simulink model "pendulumExample"  (Simulink 7.3)
settings: Solver=ode3  StartTime=0.0  StopTime=tof  FixedStep=0.01  RelTol=1e-3
InitFcn:
  | init
StopFcn:
  | plotlab
values from neighbouring files (symbols this model uses):
  Arm = [0 1;-wn^2 -2*ksi*wn]    [init.m]    (also in initPendulum2.m)
  B = [0 1]'    [init.m]    (also in initPendulum2.m = [0 0 ; 0 1])
  Brm = [0 wn^2]'    [init.m]    (also in initPendulum2.m)
  epsilon = 0.08    [init.m]    (also in initPendulum2.m)
  GammaW = 3.5    [init.m]    (also in initPendulum2.m)
  K = [1.5 0;0 1.3]    [init.m]    (also in initPendulum2.m)
  p = 10    [init.m]
  P = lyap(A',Q)    [init.m]    (also in initPendulum2.m)
  r = 1    [init.m]
  tr = [20 25]    [init.m]
  W0 = [2 -0.5 1]'    [init.m]    (also in initPendulum2.m = [2 -0.5 1 ; 0 0 0]')
  x0 = [1 1]'    [init.m]    (also in initPendulum2.m)
libraries: simulink x2, dspbuff3 x1, dspmtrx3 x1
settings Model: Creator=Alp  LastModifiedBy=alp.marangoz

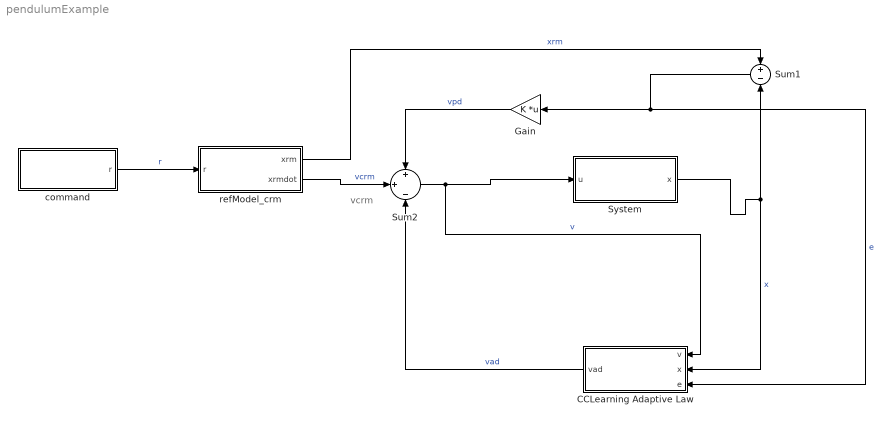
== system pendulumExample ==
  note: vcrm
  CCLearning Adaptive Law : Subsystem  TreatAsAtomicUnit=on
  Gain : Gain  Gain=K  Multiplication=Matrix(K*u)  ParameterDataType=fixdt(1, 16)  ParameterScaling=2^0  OutDataType=fixdt(1, 16)  OutScaling=2^0
  Sum1 : Sum  Inputs=+|-  OutDataType=fixdt(1, 16)  OutScaling=2^0
  Sum2 : Sum  Inputs=+|+|-  OutDataType=fixdt(1, 16)  OutScaling=2^0
  System : Subsystem  TreatAsAtomicUnit=on
  command : Subsystem
  refModel_crm : Subsystem  TreatAsAtomicUnit=on
  wires:
  command/1(r) -> refModel_crm/1(r)  "r"
  refModel_crm/1(xrm) -> Sum1/1  "xrm"
  Sum1/1 -> Gain/1, CCLearning Adaptive Law/3(e)  "e"
  Gain/1 -> Sum2/1  "vpd"
  refModel_crm/2(xrmdot) -> Sum2/2  "vcrm"
  Sum2/1 -> System/1(u), CCLearning Adaptive Law/1(v)  "v"
  CCLearning Adaptive Law/1(vad) -> Sum2/3  "vad"
  System/1(x) -> Sum1/2, CCLearning Adaptive Law/2(x)  "x"

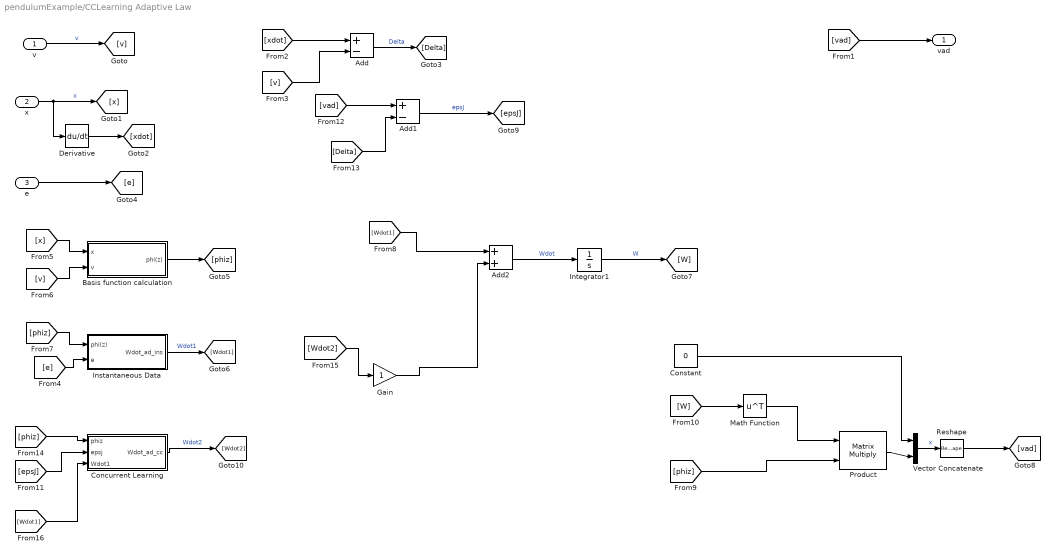
== system pendulumExample/CCLearning Adaptive Law ==
  v : Inport  OutDataType=fixdt(1, 16)  OutScaling=2^0
  x : Inport  Port=2  OutDataType=fixdt(1, 16)  OutScaling=2^0
  e : Inport  Port=3  OutDataType=fixdt(1, 16)  OutScaling=2^0
  Add : Sum  Inputs=+-  OutDataType=fixdt(1, 16)  OutScaling=2^-10
  Add1 : Sum  Inputs=+-  OutDataType=fixdt(1, 16)  OutScaling=2^-10
  Add2 : Sum  OutDataType=fixdt(1, 16)  OutScaling=2^-10
  Basis function calculation : Subsystem  TreatAsAtomicUnit=on
  Concurrent Learning : Subsystem  TreatAsAtomicUnit=on
  Constant : Constant  Value=0  OutDataType=fixdt(1, 16)  OutScaling=2^0
  Derivative : Derivative
  Gain : Gain  ParameterDataType=fixdt(1, 16)  ParameterScaling=2^0  OutDataType=fixdt(1, 16)  OutScaling=2^0
  Instantaneous Data : Subsystem  TreatAsAtomicUnit=on
  Integrator1 : Integrator  InitialCondition=W0
  Math Function : Math  Operator=transpose  OutDataType=fixdt(1, 16)  OutScaling=2^0  SaturateOnIntegerOverflow=on
  Product : Product  Multiplication=Matrix(*)  OutDataType=fixdt(1, 16)  OutScaling=2^0  RndMeth=Zero
  Reshape : Reshape  OutputDimensionality=Column vector (2-D)
  Vector Concatenate : Concatenate  Mode=Vector
  vad : Outport  OutDataType=fixdt(1, 16)  OutScaling=2^0
  wires:
  v/1 -> [v]  "v"
  [vad] -> vad/1
  x/1 -> [x], Derivative/1  "x"
  Derivative/1 -> [xdot]
  [xdot] -> Add/1
  [v] -> Add/2
  Add/1 -> [Delta]  "Delta"
  e/1 -> [e]
  [e] -> Instantaneous Data/2(e)
  [x] -> Basis function calculation/1(x)
  [v] -> Basis function calculation/2(v)
  Basis function calculation/1(phi(z)) -> [phiz]
  [phiz] -> Instantaneous Data/1(phi(z))
  Instantaneous Data/1(Wdot_ad_ins) -> [Wdot1]  "Wdot1"
  Integrator1/1 -> [W]  "W"
  [W] -> Math Function/1
  Math Function/1 -> Product/1
  [phiz] -> Product/2
  Vector Concatenate/1 -> Reshape/1  "x"
  Product/1 -> Vector Concatenate/2
  Reshape/1 -> [vad]
  Constant/1 -> Vector Concatenate/1
  [vad] -> Add1/1
  [Delta] -> Add1/2
  Add1/1 -> [epsJ]  "epsJ"
  [phiz] -> Concurrent Learning/1(phiz)
  Concurrent Learning/1(Wdot_ad_cc) -> [Wdot2]  "Wdot2"
  [epsJ] -> Concurrent Learning/2(epsj)
  [Wdot1] -> Add2/1
  Add2/1 -> Integrator1/1  "Wdot"
  [Wdot2] -> Gain/1
  [Wdot1] -> Concurrent Learning/3(Wdot1)
  Gain/1 -> Add2/2

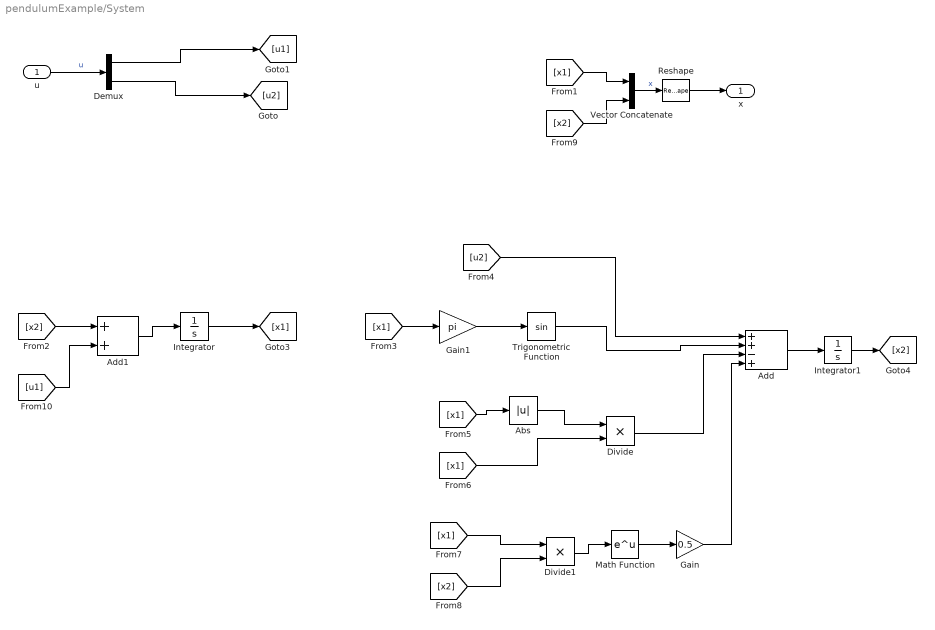
== system pendulumExample/System ==
  u : Inport  OutDataType=fixdt(1, 16)  OutScaling=2^0
  Abs : Abs  OutDataType=fixdt(1, 16)  OutScaling=2^0
  Add : Sum  Inputs=++-+  OutDataType=fixdt(1, 16)  OutScaling=2^-10
  Add1 : Sum  OutDataType=fixdt(1, 16)  OutScaling=2^-10
  Demux : Demux  Outputs=2
  Divide : Product  Inputs=**  OutDataType=fixdt(1, 16)  OutScaling=2^-10
  Divide1 : Product  Inputs=**  OutDataType=fixdt(1, 16)  OutScaling=2^-10
  Gain : Gain  Gain=0.5  ParameterDataType=fixdt(1, 16)  ParameterScaling=2^0  OutDataType=fixdt(1, 16)  OutScaling=2^0
  Gain1 : Gain  Gain=pi  ParameterDataType=fixdt(1, 16)  ParameterScaling=2^0  OutDataType=fixdt(1, 16)  OutScaling=2^0
  Integrator : Integrator  InitialCondition=x0(1,1)
  Integrator1 : Integrator  InitialCondition=x0(2,1)
  Math Function : Math  OutDataType=fixdt(1, 16)  OutScaling=2^0  SaturateOnIntegerOverflow=on
  Reshape : Reshape  OutputDimensionality=Column vector (2-D)
  Trigonometric Function : Trigonometry
  Vector Concatenate : Concatenate  Mode=Vector
  x : Outport  OutDataType=fixdt(1, 16)  OutScaling=2^0
  wires:
  Integrator/1 -> [x1]
  [x1] -> Gain1/1
  [x1] -> Abs/1
  Abs/1 -> Divide/1
  [x1] -> Divide/2
  [x1] -> Divide1/1
  [x2] -> Divide1/2
  Divide1/1 -> Math Function/1
  Math Function/1 -> Gain/1
  [u2] -> Add/1
  Trigonometric Function/1 -> Add/2
  Divide/1 -> Add/3
  Gain/1 -> Add/4
  Add/1 -> Integrator1/1
  Integrator1/1 -> [x2]
  [x1] -> Vector Concatenate/1
  [x2] -> Vector Concatenate/2
  Vector Concatenate/1 -> Reshape/1  "x"
  Reshape/1 -> x/1
  u/1 -> Demux/1  "u"
  Demux/1 -> [u1]
  Demux/2 -> [u2]
  Gain1/1 -> Trigonometric Function/1
  [x2] -> Add1/1
  Add1/1 -> Integrator/1
  [u1] -> Add1/2

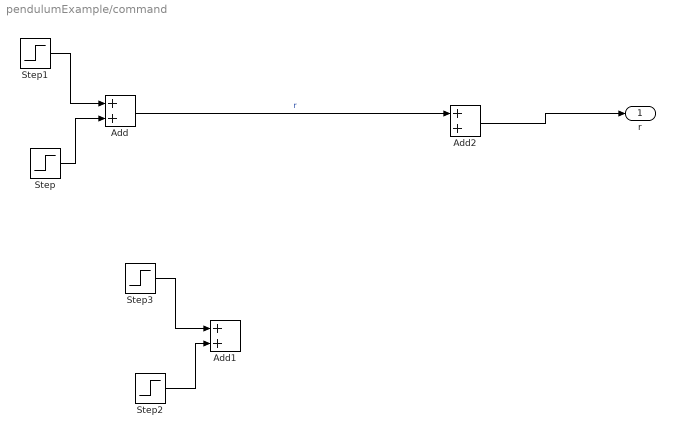
== system pendulumExample/command ==
  Add : Sum  OutDataType=fixdt(1, 16)  OutScaling=2^-10
  Add1 : Sum  OutDataType=fixdt(1, 16)  OutScaling=2^-10
  Add2 : Sum  OutDataType=fixdt(1, 16)  OutScaling=2^-10
  Step : Step  Time=tr(2)  After=-r  SampleTime=0
  Step1 : Step  Time=tr(1)  After=r  SampleTime=0
  Step2 : Step  Time=45  After=-r  SampleTime=0
  Step3 : Step  Time=40  After=r  SampleTime=0
  r : Outport
  wires:
  Step1/1 -> Add/1
  Step/1 -> Add/2
  Step3/1 -> Add1/1
  Step2/1 -> Add1/2
  Add/1 -> Add2/1  "r"
  Add2/1 -> r/1

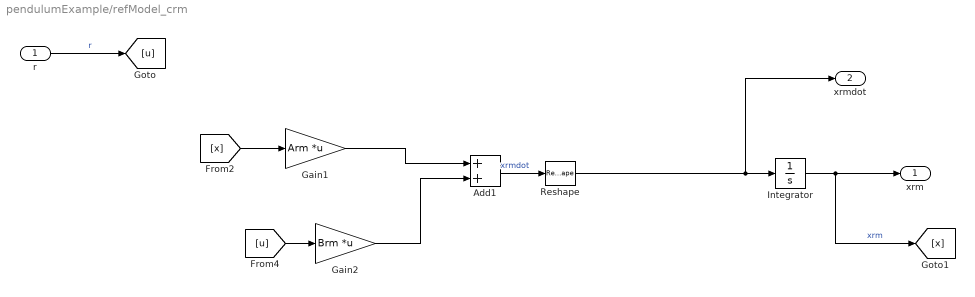
== system pendulumExample/refModel_crm ==
  r : Inport  OutDataType=fixdt(1, 16)  OutScaling=2^0
  Add1 : Sum  OutDataType=fixdt(1, 16)  OutScaling=2^-10
  Gain1 : Gain  Gain=Arm  Multiplication=Matrix(K*u)  ParameterDataType=fixdt(1, 16)  ParameterScaling=2^0  OutDataType=fixdt(1, 16)  OutScaling=2^0
  Gain2 : Gain  Gain=Brm  Multiplication=Matrix(K*u)  ParameterDataType=fixdt(1, 16)  ParameterScaling=2^0  OutDataType=fixdt(1, 16)  OutScaling=2^0
  Integrator : Integrator  InitialCondition=x0
  Reshape : Reshape  OutputDimensionality=Column vector (2-D)
  xrm : Outport  OutDataType=fixdt(1, 16)  OutScaling=2^0
  xrmdot : Outport  Port=2  OutDataType=fixdt(1, 16)  OutScaling=2^0
  wires:
  [x] -> Gain1/1
  r/1 -> [u]  "r"
  [u] -> Gain2/1
  Gain1/1 -> Add1/1
  Gain2/1 -> Add1/2
  Add1/1 -> Reshape/1  "xrmdot"
  Integrator/1 -> xrm/1, [x]  "xrm"
  Reshape/1 -> Integrator/1, xrmdot/1

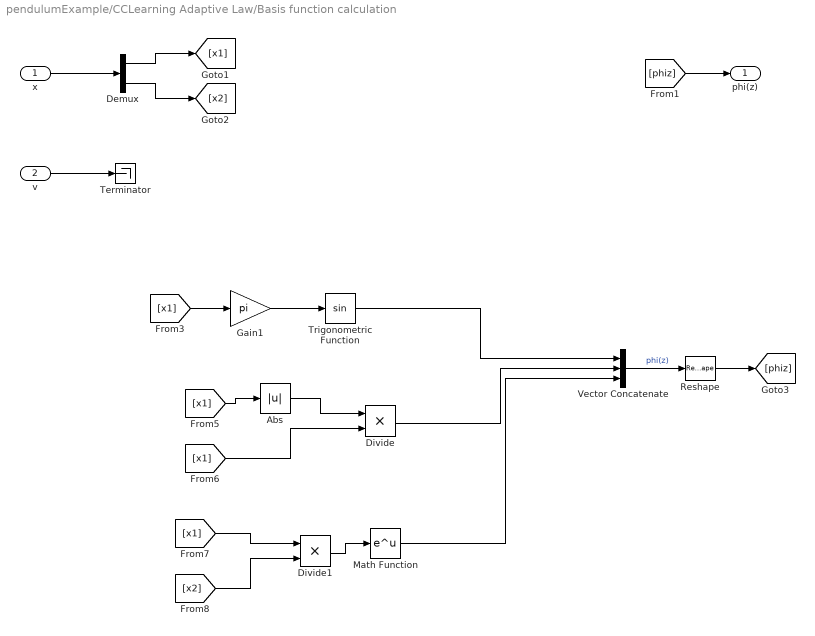
== system pendulumExample/CCLearning Adaptive Law/Basis function calculation ==
  x : Inport  OutDataType=fixdt(1, 16)  OutScaling=2^0
  v : Inport  Port=2  OutDataType=fixdt(1, 16)  OutScaling=2^0
  Abs : Abs  OutDataType=fixdt(1, 16)  OutScaling=2^0
  Demux : Demux  Outputs=2
  Divide : Product  Inputs=**  OutDataType=fixdt(1, 16)  OutScaling=2^-10
  Divide1 : Product  Inputs=**  OutDataType=fixdt(1, 16)  OutScaling=2^-10
  Gain1 : Gain  Gain=pi  ParameterDataType=fixdt(1, 16)  ParameterScaling=2^0  OutDataType=fixdt(1, 16)  OutScaling=2^0
  Math Function : Math  OutDataType=fixdt(1, 16)  OutScaling=2^0  SaturateOnIntegerOverflow=on
  Reshape : Reshape  OutputDimensionality=Column vector (2-D)
  Terminator : Terminator
  Trigonometric Function : Trigonometry
  Vector Concatenate : Concatenate  NumInputs=3  Mode=Vector
  phi(z) : Outport  OutDataType=fixdt(1, 16)  OutScaling=2^0
  wires:
  x/1 -> Demux/1
  v/1 -> Terminator/1
  [phiz] -> phi(z)/1
  [x1] -> Gain1/1
  [x1] -> Abs/1
  Abs/1 -> Divide/1
  [x1] -> Divide/2
  [x1] -> Divide1/1
  [x2] -> Divide1/2
  Divide1/1 -> Math Function/1
  Gain1/1 -> Trigonometric Function/1
  Demux/1 -> [x1]
  Demux/2 -> [x2]
  Vector Concatenate/1 -> Reshape/1  "phi(z)"
  Reshape/1 -> [phiz]
  Trigonometric Function/1 -> Vector Concatenate/1
  Divide/1 -> Vector Concatenate/2
  Math Function/1 -> Vector Concatenate/3

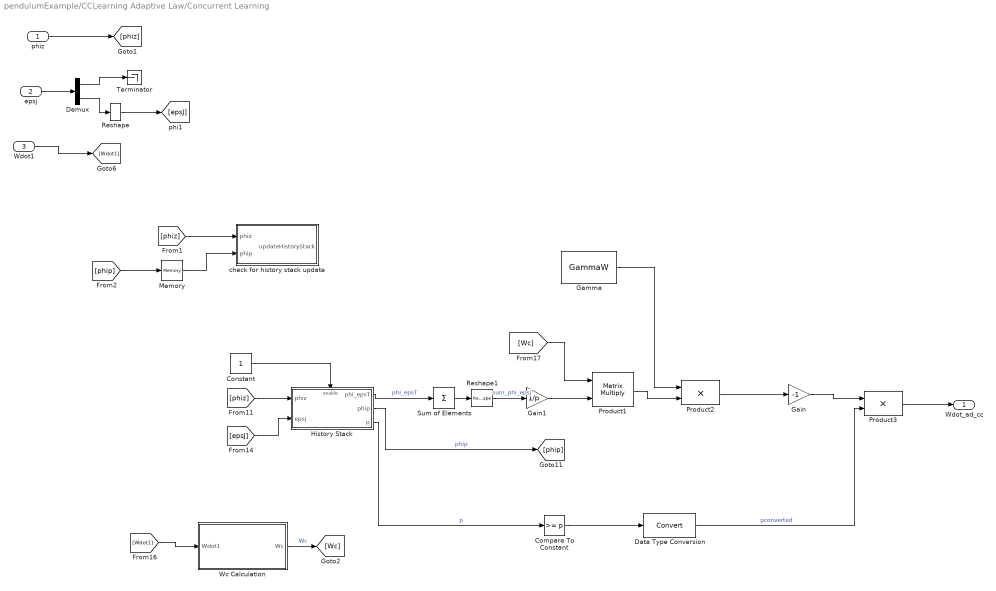
== system pendulumExample/CCLearning Adaptive Law/Concurrent Learning ==
  phiz : Inport  OutDataType=fixdt(1, 16)  OutScaling=2^0
  epsj : Inport  Port=2  OutDataType=fixdt(1, 16)  OutScaling=2^0
  Wdot1 : Inport  Port=3
  Compare To Constant : simulink/Logic and Bit Operations/Compare To Constant  SystemSampleTime=-1  relop=>=  const=p  LogicOutDataTypeMode=uint8  ZeroCross=off
  Constant : Constant  OutDataType=fixdt(1, 16)  OutScaling=2^0
  Data Type Conversion : DataTypeConversion  OutDataType=fixdt(1, 16)  OutScaling=2^0
  Demux : Demux  Outputs=2
  Gain : Gain  Gain=-1  ParameterDataType=fixdt(1, 16)  ParameterScaling=2^0  OutDataType=fixdt(1, 16)  OutScaling=2^0
  Gain1 : Gain  Gain=1/p  ParameterDataType=fixdt(1, 16)  ParameterScaling=2^0  OutDataType=fixdt(1, 16)  OutScaling=2^0
  Gamma : Constant  Value=GammaW  VectorParams1D=off  OutDataType=fixdt(1, 16)  OutScaling=2^0
  History Stack : Subsystem  TreatAsAtomicUnit=on
  Memory : Memory
  Product1 : Product  Multiplication=Matrix(*)  OutDataType=fixdt(1, 16)  OutScaling=2^0  RndMeth=Zero
  Product2 : Product  OutDataType=fixdt(1, 16)  OutScaling=2^0  RndMeth=Zero
  Product3 : Product  OutDataType=fixdt(1, 16)  OutScaling=2^0  RndMeth=Zero
  Reshape : Reshape  OutputDimensionality=Column vector (2-D)
  Reshape1 : Reshape  OutputDimensionality=Column vector (2-D)
  Sum of Elements : Sum  Inputs=+  CollapseMode=Specified dimension  OutDataType=fixdt(1, 16)  OutScaling=2^-10
  Terminator : Terminator
  Wc Calculation : Subsystem
  check for history stack update : Subsystem  TreatAsAtomicUnit=on
  Wdot_ad_cc : Outport  OutDataType=fixdt(1, 16)  OutScaling=2^0
  wires:
  [phiz] -> History Stack/1(phiz)
  [epsJ] -> History Stack/2(epsj)
  History Stack/1(phi_epsT) -> Sum of Elements/1  "phi_epsT"
  Gamma/1 -> Product2/1
  Product2/1 -> Gain/1
  History Stack/2(phip) -> [phip]  "phip"
  phiz/1 -> [phiz]
  Demux/1 -> Terminator/1
  Demux/2 -> Reshape/1
  epsj/1 -> Demux/1
  Reshape/1 -> [epsJ]
  [phiz] -> check for history stack update/1(phiz)
  [phip] -> Memory/1
  Memory/1 -> check for history stack update/2(phip)
  Sum of Elements/1 -> Reshape1/1
  Wdot1/1 -> [Wdot1]
  [Wdot1] -> Wc Calculation/1(Wdot1)
  Wc Calculation/1(Wc) -> [Wc]  "Wc"
  Reshape1/1 -> Gain1/1  "sum_phi_epsj"
  Product1/1 -> Product2/2
  [Wc] -> Product1/1
  Gain1/1 -> Product1/2
  History Stack/3(p) -> Compare To Constant/1  "p"
  Compare To Constant/1 -> Data Type Conversion/1
  Gain/1 -> Product3/1
  Data Type Conversion/1 -> Product3/2  "pconverted"
  Product3/1 -> Wdot_ad_cc/1
  Constant/1 -> History Stack/Enable

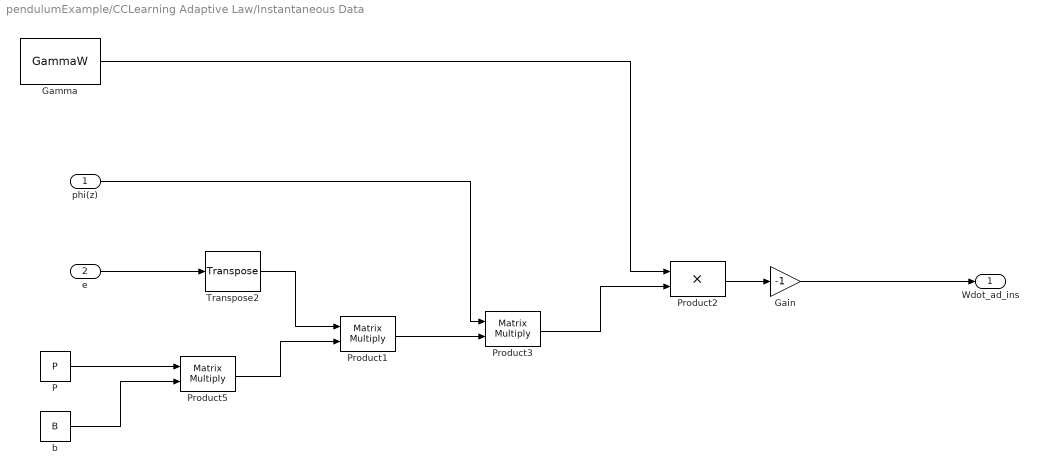
== system pendulumExample/CCLearning Adaptive Law/Instantaneous Data ==
  phi(z) : Inport  OutDataType=fixdt(1, 16)  OutScaling=2^0
  e : Inport  Port=2  OutDataType=fixdt(1, 16)  OutScaling=2^0
  Gain : Gain  Gain=-1  ParameterDataType=fixdt(1, 16)  ParameterScaling=2^0  OutDataType=fixdt(1, 16)  OutScaling=2^0
  Gamma : Constant  Value=GammaW  VectorParams1D=off  OutDataType=fixdt(1, 16)  OutScaling=2^0
  P : Constant  Value=P  VectorParams1D=off  OutDataType=fixdt(1, 16)  OutScaling=2^0
  Product1 : Product  Multiplication=Matrix(*)  OutDataType=fixdt(1, 16)  OutScaling=2^0  RndMeth=Zero
  Product2 : Product  OutDataType=fixdt(1, 16)  OutScaling=2^0  RndMeth=Zero
  Product3 : Product  Multiplication=Matrix(*)  OutDataType=fixdt(1, 16)  OutScaling=2^0  RndMeth=Zero
  Product5 : Product  Multiplication=Matrix(*)  OutDataType=fixdt(1, 16)  OutScaling=2^0  RndMeth=Zero
  Transpose2 : dspmtrx3/Transpose  SystemSampleTime=-1  Hermitian=off  overflowFlag=off
  b : Constant  Value=B  VectorParams1D=off  OutDataType=fixdt(1, 16)  OutScaling=2^0
  Wdot_ad_ins : Outport  OutDataType=fixdt(1, 16)  OutScaling=2^0
  wires:
  P/1 -> Product5/1
  b/1 -> Product5/2
  e/1 -> Transpose2/1
  Transpose2/1 -> Product1/1
  Product5/1 -> Product1/2
  phi(z)/1 -> Product3/1
  Product1/1 -> Product3/2
  Gamma/1 -> Product2/1
  Product3/1 -> Product2/2
  Product2/1 -> Gain/1
  Gain/1 -> Wdot_ad_ins/1

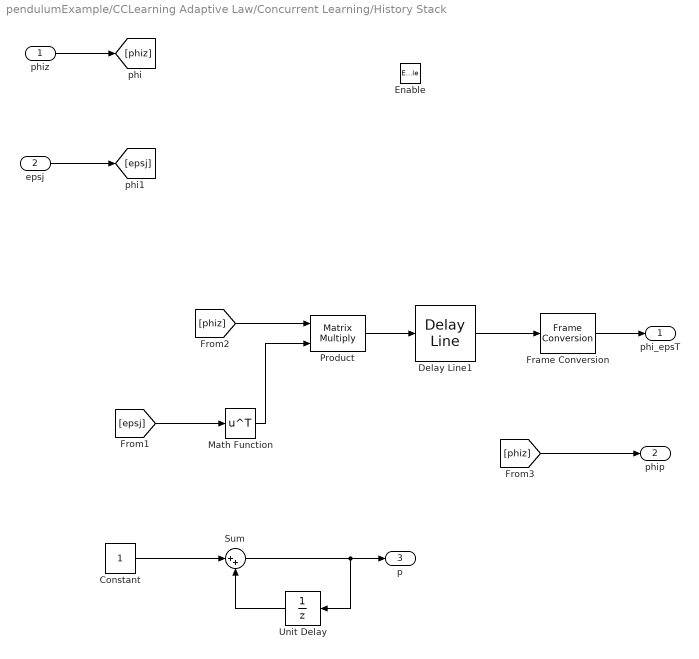
== system pendulumExample/CCLearning Adaptive Law/Concurrent Learning/History Stack ==
  phiz : Inport  OutDataType=fixdt(1, 16)  OutScaling=2^0
  epsj : Inport  Port=2  OutDataType=fixdt(1, 16)  OutScaling=2^0
  Enable : EnablePort
  Constant : Constant  OutDataType=fixdt(1, 16)  OutScaling=2^0
  Delay Line1 : dspbuff3/Delay Line  siz=p  ic=0  directfeed=on  enable_output=off  hold_output=off
  Frame Conversion : FrameConversion  OutFrame=Sample-based
  Math Function : Math  Operator=transpose  OutDataType=fixdt(1, 16)  OutScaling=2^0  SaturateOnIntegerOverflow=on
  Product : Product  Multiplication=Matrix(*)  OutDataType=fixdt(1, 16)  OutScaling=2^0  RndMeth=Zero
  Sum : Sum  Inputs=|++  OutDataType=fixdt(1, 16)  OutScaling=2^0
  Unit Delay : UnitDelay  SampleTime=-1
  phi_epsT : Outport  OutDataType=fixdt(1, 16)  OutScaling=2^0
  phip : Outport  Port=2  OutDataType=fixdt(1, 16)  OutScaling=2^0
  p : Outport  Port=3  OutDataType=fixdt(1, 16)  OutScaling=2^0
  wires:
  [phiz] -> Product/1
  phiz/1 -> [phiz]
  [epsj] -> Math Function/1
  Product/1 -> Delay Line1/1
  Delay Line1/1 -> Frame Conversion/1
  [phiz] -> phip/1
  Math Function/1 -> Product/2
  epsj/1 -> [epsj]
  Frame Conversion/1 -> phi_epsT/1
  Constant/1 -> Sum/1
  Sum/1 -> p/1, Unit Delay/1
  Unit Delay/1 -> Sum/2

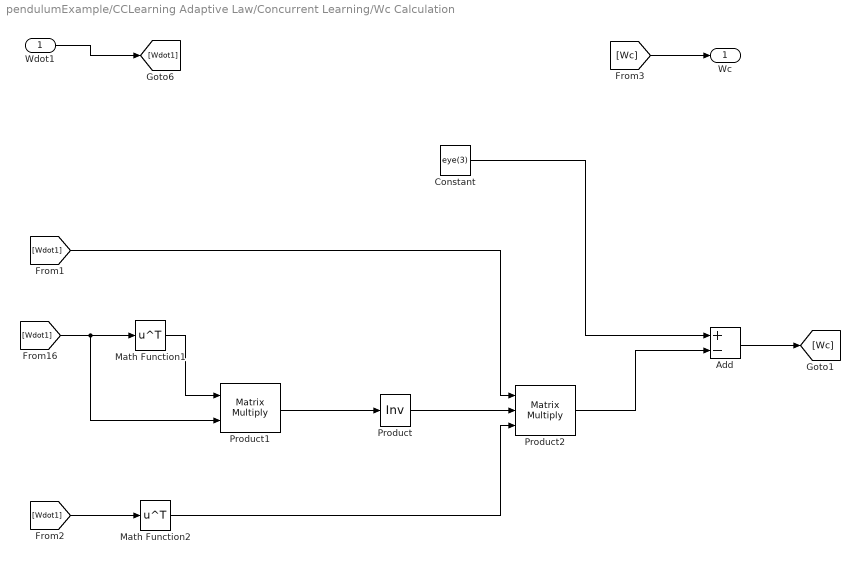
== system pendulumExample/CCLearning Adaptive Law/Concurrent Learning/Wc Calculation ==
  Wdot1 : Inport
  Add : Sum  Inputs=+-  OutDataType=fixdt(1, 16)  OutScaling=2^-10
  Constant : Constant  Value=eye(3)  OutDataType=fixdt(1, 16)  OutScaling=2^0
  Math Function1 : Math  Operator=transpose  OutDataType=fixdt(1, 16)  OutScaling=2^0  SaturateOnIntegerOverflow=on
  Math Function2 : Math  Operator=transpose  OutDataType=fixdt(1, 16)  OutScaling=2^0  SaturateOnIntegerOverflow=on
  Product : Product  Inputs=/  Multiplication=Matrix(*)  OutDataType=fixdt(1, 16)  OutScaling=2^0  RndMeth=Zero
  Product1 : Product  Multiplication=Matrix(*)  OutDataType=fixdt(1, 16)  OutScaling=2^0  RndMeth=Zero
  Product2 : Product  Inputs=***  Multiplication=Matrix(*)  OutDataType=fixdt(1, 16)  OutScaling=2^0  RndMeth=Zero
  Wc : Outport
  wires:
  [Wdot1] -> Math Function1/1, Product1/2
  Math Function1/1 -> Product1/1
  Product1/1 -> Product/1
  Wdot1/1 -> [Wdot1]
  [Wdot1] -> Math Function2/1
  [Wdot1] -> Product2/1
  Product/1 -> Product2/2
  Math Function2/1 -> Product2/3
  Constant/1 -> Add/1
  Add/1 -> [Wc]
  [Wc] -> Wc/1
  Product2/1 -> Add/2

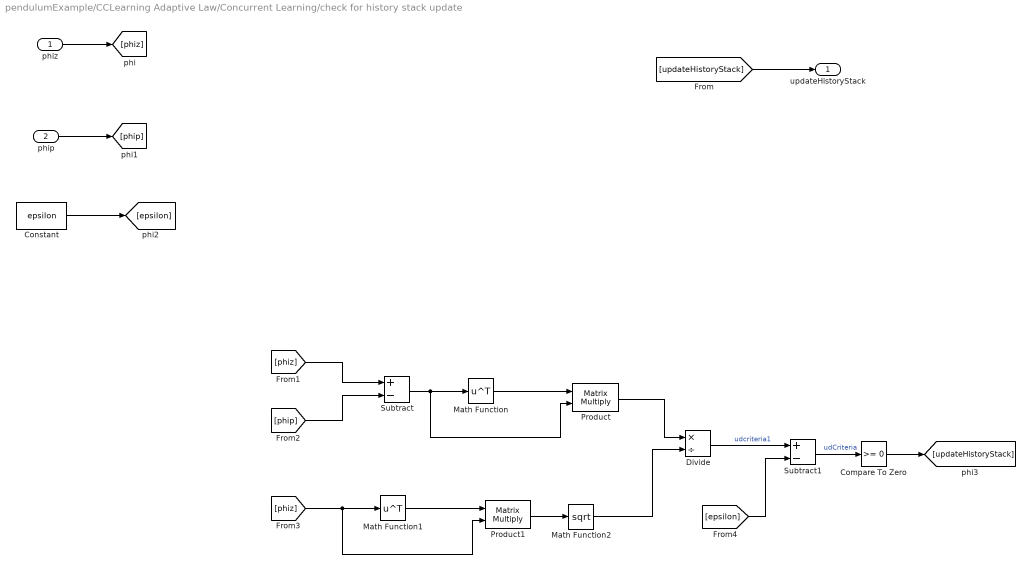
== system pendulumExample/CCLearning Adaptive Law/Concurrent Learning/check for history stack update ==
  phiz : Inport  OutDataType=fixdt(1, 16)  OutScaling=2^0
  phip : Inport  Port=2  OutDataType=fixdt(1, 16)  OutScaling=2^0
  Compare To Zero : simulink/Logic and Bit Operations/Compare To Zero  SystemSampleTime=-1  relop=>=  LogicOutDataTypeMode=uint8  ZeroCross=off
  Constant : Constant  Value=epsilon  OutDataType=fixdt(1, 16)  OutScaling=2^0
  Divide : Product  Inputs=*/  OutDataType=fixdt(1, 16)  OutScaling=2^-10
  Math Function : Math  Operator=transpose  OutDataType=fixdt(1, 16)  OutScaling=2^0  SaturateOnIntegerOverflow=on
  Math Function1 : Math  Operator=transpose  OutDataType=fixdt(1, 16)  OutScaling=2^0  SaturateOnIntegerOverflow=on
  Math Function2 : Math  Operator=sqrt  OutDataType=fixdt(1, 16)  OutScaling=2^0  SaturateOnIntegerOverflow=on
  Product : Product  Multiplication=Matrix(*)  OutDataType=fixdt(1, 16)  OutScaling=2^0  RndMeth=Zero
  Product1 : Product  Multiplication=Matrix(*)  OutDataType=fixdt(1, 16)  OutScaling=2^0  RndMeth=Zero
  Subtract : Sum  Inputs=+-  OutDataType=fixdt(1, 16)  OutScaling=2^-10
  Subtract1 : Sum  Inputs=+-  OutDataType=fixdt(1, 16)  OutScaling=2^-10
  updateHistoryStack : Outport  OutDataType=fixdt(1, 16)  OutScaling=2^0
  wires:
  phip/1 -> [phip]
  phiz/1 -> [phiz]
  [updateHistoryStack] -> updateHistoryStack/1
  Constant/1 -> [epsilon]
  [phiz] -> Subtract/1
  [phip] -> Subtract/2
  Subtract/1 -> Math Function/1, Product/2
  Math Function/1 -> Product/1
  [phiz] -> Product1/2, Math Function1/1
  Math Function1/1 -> Product1/1
  Product1/1 -> Math Function2/1
  Product/1 -> Divide/1
  Divide/1 -> Subtract1/1  "udcriteria1"
  [epsilon] -> Subtract1/2
  Subtract1/1 -> Compare To Zero/1  "udCriteria"
  Compare To Zero/1 -> [updateHistoryStack]
  Math Function2/1 -> Divide/2
